simulink model "SSC_Robust_LQR"  (R2024b)
settings: Solver=VariableStepAuto  StartTime=0.0  StopTime=10.0  RelTol=1e-3
undefined symbols (not defined in the file or in its folder): drv, rpm2rads, ssc_LQR_aug
settings Model: Creator=llp  LastModifiedBy=llp

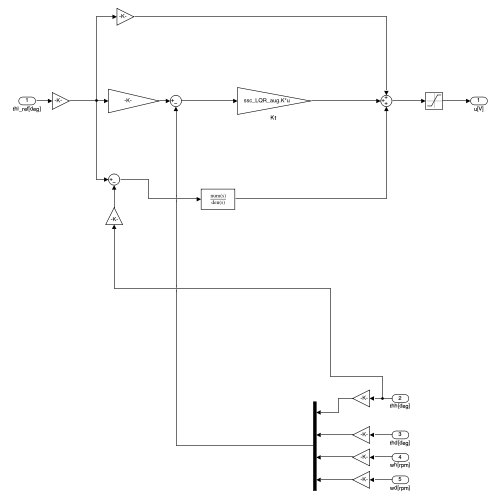
[thumbnail: Simulink's stored preview of the top-level diagram]
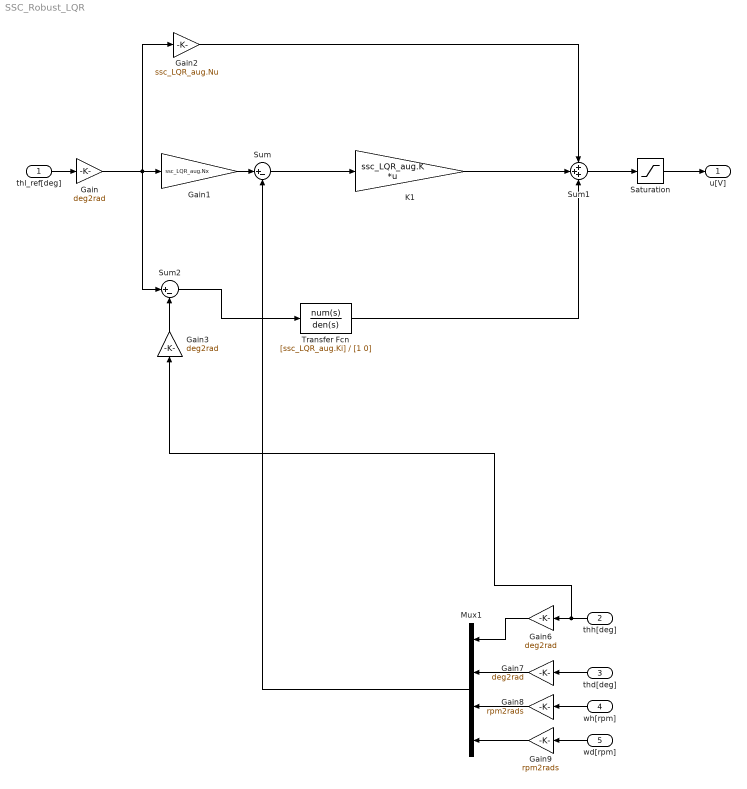
== system SSC_Robust_LQR ==
  thl_ref[deg] : Inport
  thh[deg] : Inport  Port=2
  thd[deg] : Inport  Port=3
  wh[rpm] : Inport  Port=4
  wd[rpm] : Inport  Port=5
  Gain{,3,6..7} (4 alike) : Gain  Gain=deg2rad
  Gain1 : Gain  Gain=ssc_LQR_aug.Nx
  Gain2 : Gain  Gain=ssc_LQR_aug.Nu
  Gain8 : Gain  Gain=rpm2rads
  Gain9 : Gain  Gain=rpm2rads
  K1 : Gain  Gain=ssc_LQR_aug.K  Multiplication=Matrix(K*u)
  Mux1 : Mux
  Saturation : Saturate  UpperLimit=drv.outmax  LowerLimit=-drv.outmax
  Sum : Sum  Inputs=|+-
  Sum1 : Sum  Inputs=+++
  Sum2 : Sum  Inputs=|+-
  Transfer Fcn : TransferFcn  Numerator=[ssc_LQR_aug.Ki]  Denominator=[1 0]
  u[V] : Outport
  wires:
  thl_ref[deg]/1 -> Gain/1
  Gain1/1 -> Sum/1
  thh[deg]/1 -> Gain3/1, Gain6/1
  Sum1/1 -> Saturation/1
  Gain3/1 -> Sum2/2
  Gain/1 -> Gain1/1, Sum2/1, Gain2/1
  K1/1 -> Sum1/2
  Sum2/1 -> Transfer Fcn/1
  Gain2/1 -> Sum1/1
  Sum/1 -> K1/1
  Saturation/1 -> u[V]/1
  Gain9/1 -> Mux1/4
  thd[deg]/1 -> Gain7/1
  wh[rpm]/1 -> Gain8/1
  Gain7/1 -> Mux1/2
  Gain6/1 -> Mux1/1
  wd[rpm]/1 -> Gain9/1
  Gain8/1 -> Mux1/3
  Mux1/1 -> Sum/2
  Transfer Fcn/1 -> Sum1/3
